simulink model "Test_Arithmetic_Operation"  (Simulink 8.1)
settings: Solver=ode45  StartTime=0.0  StopTime=10.0  RelTol=1e-3
libraries: Arithmetic_Operations_Lib x6, commutil2 x2
settings Model: Creator=uzivatel  LastModifiedBy=uzivatel
settings DataIOCC: SignalLoggingSaveFormat=Dataset
settings OptimizationCC: ExpressionDepthLimit=128
settings DebuggingCC: FcnCallInpInsideContextMsg=EnableAllAsError
settings GRTTargetCC: CombineOutputUpdateFcns=on  GRTInterface=off

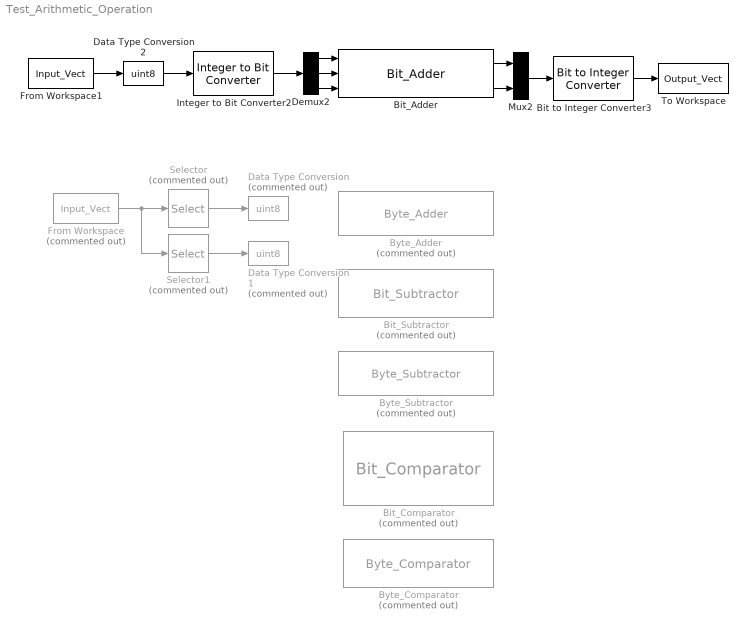
== system Test_Arithmetic_Operation ==
  Bit to Integer Converter3 : commutil2/Bit to Integer Converter  nbits=2  bitOrder=MSB first  signedOutputValues=Unsigned  outDtype=uint8  outDtypeSigned=Inherit via internal rule
  Bit_Adder : Arithmetic_Operations_Lib/Arithmetic_Operations_Lib/Bit_Adder
  Bit_Comparator : Arithmetic_Operations_Lib/Arithmetic_Operations_Lib/Bit_Comparator  Commented=on
  Bit_Subtractor : Arithmetic_Operations_Lib/Arithmetic_Operations_Lib/Bit_Subtractor  Commented=on
  Byte_Adder : Arithmetic_Operations_Lib/Arithmetic_Operations_Lib/Byte_Adder  Commented=on
  Byte_Comparator : Arithmetic_Operations_Lib/Arithmetic_Operations_Lib/Byte_Comparator  Commented=on
  Byte_Subtractor : Arithmetic_Operations_Lib/Arithmetic_Operations_Lib/Byte_Subtractor  Commented=on
  Data Type Conversion : DataTypeConversion  Commented=on  OutDataTypeStr=uint8
  Data Type Conversion1 : DataTypeConversion  Commented=on  OutDataTypeStr=uint8
  Data Type Conversion2 : DataTypeConversion  OutDataTypeStr=uint8
  Demux2 : Demux  Outputs=3
  From Workspace : FromWorkspace  Commented=on  VariableName=Input_Vect  SampleTime=1  Interpolate=off  OutputAfterFinalValue=Holding final value
  From Workspace1 : FromWorkspace  VariableName=Input_Vect  SampleTime=1  Interpolate=off  OutputAfterFinalValue=Holding final value
  Integer to Bit Converter2 : commutil2/Integer to Bit Converter  nbits=3  signedInputValues=Unsigned  bitOrder=MSB first  outDtype=boolean
  Mux2 : Mux  Inputs=2
  Selector : Selector  Commented=on  IndexMode=Zero-based  InputPortWidth=2  SampleTime=1  IndexOptions=Index vector (dialog)  Indices=0  OutputSizes=1
  Selector1 : Selector  Commented=on  IndexMode=Zero-based  InputPortWidth=2  SampleTime=1  IndexOptions=Index vector (dialog)  Indices=1  OutputSizes=1
  To Workspace : ToWorkspace  VariableName=Output_Vect  SampleTime=1
  wires:
  From Workspace/1 -> Selector1/1, Selector/1
  Selector/1 -> Data Type Conversion/1
  Selector1/1 -> Data Type Conversion1/1
  From Workspace1/1 -> Data Type Conversion2/1
  Data Type Conversion2/1 -> Integer to Bit Converter2/1
  Integer to Bit Converter2/1 -> Demux2/1
  Demux2/1 -> Bit_Adder/1
  Demux2/2 -> Bit_Adder/2
  Demux2/3 -> Bit_Adder/3
  Bit_Adder/1 -> Mux2/1
  Bit_Adder/2 -> Mux2/2
  Mux2/1 -> Bit to Integer Converter3/1
  Bit to Integer Converter3/1 -> To Workspace/1
